simulink model "Inverted_pendulum_Simulink_Block"  (R2017a)
settings: Solver=VariableStepAuto  StartTime=0.0  StopTime=10.0  RelTol=1e-3
values from neighbouring files (symbols this model uses):
  b = 0.1    [Inverted_Pendulum_State_Space.m]    (also in Inverted_Pendulum_Transfer_Function.m)
  I = 0.006    [Inverted_Pendulum_State_Space.m]    (also in Inverted_Pendulum_Transfer_Function.m)
  L = 0.3    [Inverted_Pendulum_State_Space.m]    (also in Inverted_Pendulum_Transfer_Function.m)
  m = 0.2    [Inverted_Pendulum_State_Space.m]    (also in Inverted_Pendulum_Transfer_Function.m)
  M = 0.5    [Inverted_Pendulum_State_Space.m]    (also in Inverted_Pendulum_Transfer_Function.m)
settings Model: Creator=Majed  LastModifiedBy=Majed
settings SolverCC: AlgebraicLoopSolver=LineSearch

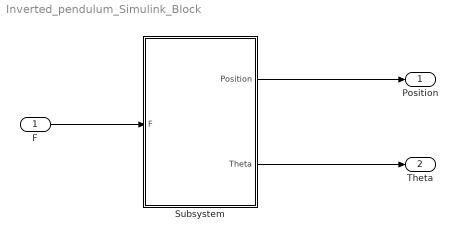
== system Inverted_pendulum_Simulink_Block ==
  F : Inport
  Subsystem : Subsystem
  Position : Outport
  Theta : Outport  Port=2
  wires:
  F/1 -> Subsystem/1(F)
  Subsystem/1(Position) -> Position/1
  Subsystem/2(Theta) -> Theta/1

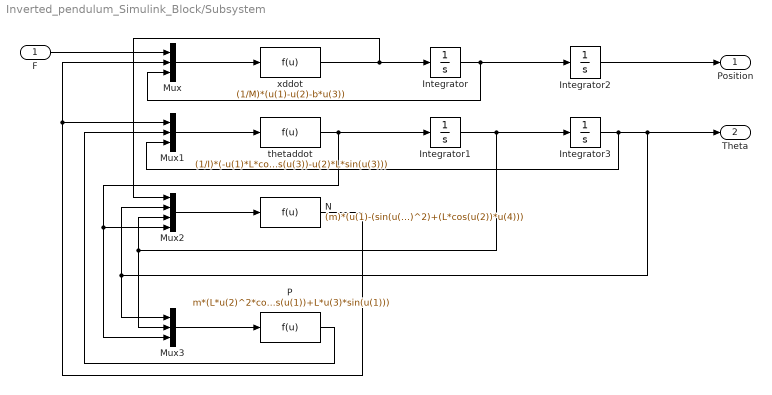
== system Inverted_pendulum_Simulink_Block/Subsystem ==
  F : Inport
  Integrator : Integrator  ContinuousStateAttributes='xdot'
  Integrator1 : Integrator  InitialCondition=pi  ContinuousStateAttributes='Thetadot'
  Integrator2 : Integrator  ContinuousStateAttributes='x'
  Integrator3 : Integrator  InitialCondition=pi  ContinuousStateAttributes='Theta'
  Mux : Mux  Inputs=3
  Mux1 : Mux  Inputs=3
  Mux2 : Mux
  Mux3 : Mux  Inputs=3
  N : Fcn  Expr=(m)*(u(1)-(sin(u(2))*L*u(3)^2)+(L*cos(u(2))*u(4)))
  P : Fcn  Expr=m*(L*u(2)^2*cos(u(1))+L*u(3)*sin(u(1)))
  thetaddot : Fcn  Expr=(1/I)*(-u(1)*L*cos(u(3))-u(2)*L*sin(u(3)))
  xddot : Fcn  Expr=(1/M)*(u(1)-u(2)-b*u(3))
  Position : Outport
  Theta : Outport  Port=2
  wires:
  Mux1/1 -> thetaddot/1
  Mux/1 -> xddot/1
  thetaddot/1 -> Mux2/4, Mux3/3, Integrator1/1
  Mux3/1 -> P/1
  Mux2/1 -> N/1
  xddot/1 -> Mux2/1, Integrator/1
  Integrator/1 -> Mux/3, Integrator2/1
  N/1 -> Mux/2, Mux1/1
  F/1 -> Mux/1
  Integrator2/1 -> Position/1
  Integrator1/1 -> Mux2/3, Mux3/2, Integrator3/1
  P/1 -> Mux1/2
  Integrator3/1 -> Mux1/3, Theta/1, Mux3/1, Mux2/2
